simulink model "surgicalControl_Shared_memory_q_2015b"  (R2015b)
settings: Solver=FixedStepAuto  SolverMode=SingleTasking  StartTime=0.0  StopTime=inf  FixedStep=1/100  RelTol=1e-3
libraries: simulink x3, matlabGenericSHM_Block x1
settings Model: Creator=daniel  LastModifiedBy=Bogdan
settings DataIOCC: LimitDataPoints=off
settings DebuggingCC: AllowSymbolicDim=on  SFUnexpectedBacktrackingDiag=error  SFNoUnconditionalDefaultTransitionDiag=error
settings ModelReferenceCC: PropagateSignalLabelsOutOfModel=on
settings GRTTargetCC: TargetLangStandard=C99 (ISO)
settings ConfigComp: CovMetricSettings=dwe  CovHtmlReporting=off  CovSaveCumulativeToWorkspaceVar=off  CovSaveSingleToWorkspaceVar=off  CovModelRefEnable=Off  CovExternalEMLEnable=on

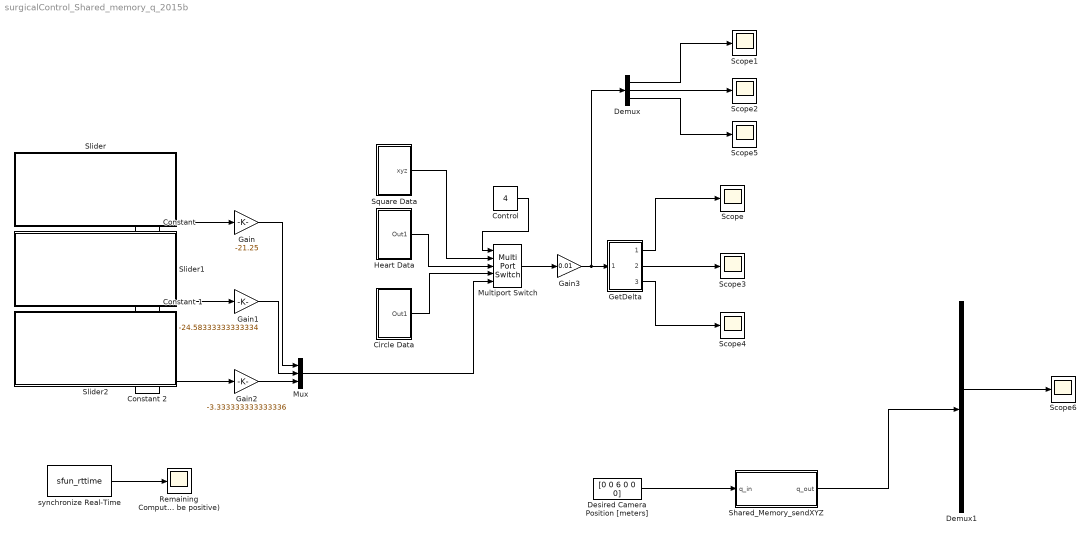
== system surgicalControl_Shared_memory_q_2015b ==
  " GetDelta " : Subsystem
  " Constant " : Constant
  " Constant 1" : Constant
  " Constant 2" : Constant
  "Circle Data " : Subsystem
  "Control " : Constant  Value=4
  Demux : Demux  Outputs=3
  Demux1 : Demux  Outputs=6
  Desired Camera Position [meters] : Constant  Value=[0 0 6 0 0 0]  OutDataTypeStr=single
  Gain : Gain  Gain=-21.25
  Gain1 : Gain  Gain=-24.58333333333334
  Gain2 : Gain  Gain=-3.333333333333336
  Gain3 : Gain  Gain=0.01
  "Heart Data " : Subsystem
  Multiport Switch : MultiPortSwitch  Inputs=4
  Mux : Mux  Inputs=3
  Remaining Computation Time (must be positive) : Scope
  Scope{,1..6} (7 alike) : Scope
  Shared_Memory_sendXYZ : Subsystem  mask{ID1=4}
  Slider : Subsystem  DialogController=hmiCreateDDGDialog  IsWebBlock=on  mask(MWDashboardBlock){webBlockId=4f94596f-dd6d-4e5e-bddc-7a8d913927f9, webBlockType=slider, ShowInLibBrowser=on, ShowInitialText=on, HMISrcModelName=surgicalControl_Shared_memory_q_2015b}
      mask prompts: webBlockId "WebBlock Id"; webBlockType "WebBlock Type"; HMISrcModelName "Source Model"
      mask help: SimulinkHMI:dialogs:SliderDialogDesc
      mask Help: helpview([docroot '/mapfiles/simulink.map'], 'hmi_slider')
      mask Display:
      | if strcmp(get_param(bdroot(gcb),'BlockDiagramType'), 'library')
      |     image([(matlabroot) '/toolbox/simulink/hmi/icons/Slider.png']);
      | end
  Slider1 : Subsystem  DialogController=hmiCreateDDGDialog  IsWebBlock=on  mask(MWDashboardBlock){webBlockId=8aa996ad-7cd4-40fc-9a04-6a85939aea5d, webBlockType=slider, ShowInLibBrowser=on, ShowInitialText=on, HMISrcModelName=surgicalControl_Shared_memory_q_2015b}
      mask prompts: webBlockId "WebBlock Id"; webBlockType "WebBlock Type"; HMISrcModelName "Source Model"
      mask help: SimulinkHMI:dialogs:SliderDialogDesc
      mask Help: helpview([docroot '/mapfiles/simulink.map'], 'hmi_slider')
      mask Display:
      | if strcmp(get_param(bdroot(gcb),'BlockDiagramType'), 'library')
      |     image([(matlabroot) '/toolbox/simulink/hmi/icons/Slider.png']);
      | end
  Slider2 : Subsystem  DialogController=hmiCreateDDGDialog  IsWebBlock=on  mask(MWDashboardBlock){webBlockId=1ddf6fd9-0225-4881-82ca-a25e179e2ab9, webBlockType=slider, ShowInLibBrowser=on, ShowInitialText=on, HMISrcModelName=surgicalControl_Shared_memory_q_2015b}
      mask prompts: webBlockId "WebBlock Id"; webBlockType "WebBlock Type"; HMISrcModelName "Source Model"
      mask help: SimulinkHMI:dialogs:SliderDialogDesc
      mask Help: helpview([docroot '/mapfiles/simulink.map'], 'hmi_slider')
      mask Display:
      | if strcmp(get_param(bdroot(gcb),'BlockDiagramType'), 'library')
      |     image([(matlabroot) '/toolbox/simulink/hmi/icons/Slider.png']);
      | end
  "Square Data " : Subsystem
  synchronize Real-Time : S-Function  FunctionName=sfun_rttime  Parameters=1  SFunctionDeploymentMode=off  EnableBusSupport=off
  wires:
  " GetDelta "/1(Out1) -> Scope/1
  " GetDelta "/2(Out2) -> Scope3/1
  " GetDelta "/3(Out3) -> Scope4/1
  Multiport Switch/1 -> Gain3/1
  "Square Data "/1(xyz) -> Multiport Switch/2
  "Control "/1 -> Multiport Switch/1
  " Constant "/1 -> Gain/1
  " Constant 1"/1 -> Gain1/1
  " Constant 2"/1 -> Gain2/1
  Gain/1 -> Mux/1
  Gain1/1 -> Mux/2
  Gain2/1 -> Mux/3
  Mux/1 -> Multiport Switch/5
  "Heart Data "/1(Out1) -> Multiport Switch/3
  "Circle Data "/1(Out1) -> Multiport Switch/4
  Demux/2 -> Scope2/1
  Demux/1 -> Scope1/1
  Demux/3 -> Scope5/1
  synchronize Real-Time/1 -> Remaining Computation Time (must be positive)/1
  Gain3/1 -> Demux/1, " GetDelta "/1(In1)
  Shared_Memory_sendXYZ/1(q_out) -> Demux1/1
  Desired Camera Position [meters]/1 -> Shared_Memory_sendXYZ/1(q_in)
  Demux1/3 -> Scope6/1

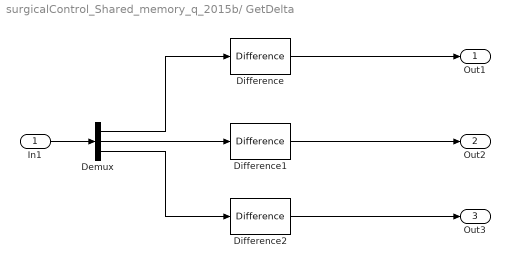
== system surgicalControl_Shared_memory_q_2015b/ GetDelta  ==
  In1 : Inport
  Demux : Demux  Outputs=3
  Difference : simulink/Discrete/Difference  ICPrevInput=0  OutMin=[]  OutMax=[]  OutDataType=fixdt(1, 16)  OutScaling=2^-10  DoSatur=off
  Difference1 : simulink/Discrete/Difference  ICPrevInput=0  OutMin=[]  OutMax=[]  OutDataType=fixdt(1, 16)  OutScaling=2^-10  DoSatur=off
  Difference2 : simulink/Discrete/Difference  ICPrevInput=0  OutMin=[]  OutMax=[]  OutDataType=fixdt(1, 16)  OutScaling=2^-10  DoSatur=off
  Out1 : Outport
  Out2 : Outport  Port=2
  Out3 : Outport  Port=3
  wires:
  Difference1/1 -> Out2/1
  Difference/1 -> Out1/1
  Difference2/1 -> Out3/1
  In1/1 -> Demux/1
  Demux/1 -> Difference/1
  Demux/2 -> Difference1/1
  Demux/3 -> Difference2/1

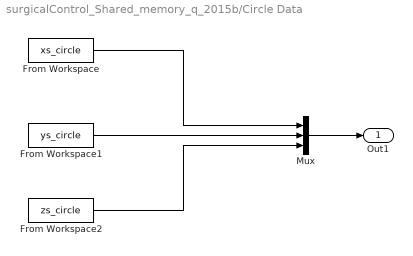
== system surgicalControl_Shared_memory_q_2015b/Circle Data  ==
  From Workspace : FromWorkspace  VariableName=xs_circle  SampleTime=1
  From Workspace1 : FromWorkspace  VariableName=ys_circle  SampleTime=1
  From Workspace2 : FromWorkspace  VariableName=zs_circle  SampleTime=1
  Mux : Mux  Inputs=3
  Out1 : Outport
  wires:
  From Workspace/1 -> Mux/1
  From Workspace2/1 -> Mux/3
  Mux/1 -> Out1/1
  From Workspace1/1 -> Mux/2

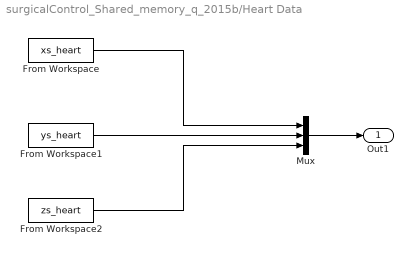
== system surgicalControl_Shared_memory_q_2015b/Heart Data  ==
  From Workspace : FromWorkspace  VariableName=xs_heart  SampleTime=1
  From Workspace1 : FromWorkspace  VariableName=ys_heart  SampleTime=1
  From Workspace2 : FromWorkspace  VariableName=zs_heart  SampleTime=1
  Mux : Mux  Inputs=3
  Out1 : Outport
  wires:
  From Workspace/1 -> Mux/1
  From Workspace2/1 -> Mux/3
  Mux/1 -> Out1/1
  From Workspace1/1 -> Mux/2

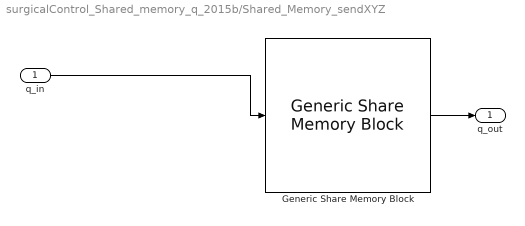
== system surgicalControl_Shared_memory_q_2015b/Shared_Memory_sendXYZ ==
  q_in : Inport
  Generic Share Memory Block : matlabGenericSHM_Block/Generic Share Memory Block  nombre='EyeRob'  dispositivo=ID1  vecE=[6]  vecS=[6]  tipoE=['f']  tipoS=['f']
  q_out : Outport
  wires:
  q_in/1 -> Generic Share Memory Block/1
  Generic Share Memory Block/1 -> q_out/1

== system surgicalControl_Shared_memory_q_2015b/Slider ==

== system surgicalControl_Shared_memory_q_2015b/Slider1 ==

== system surgicalControl_Shared_memory_q_2015b/Slider2 ==

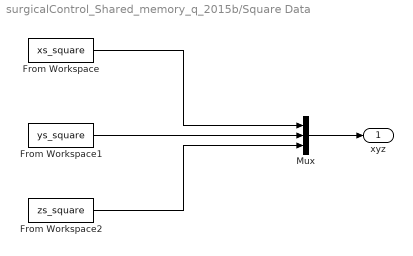
== system surgicalControl_Shared_memory_q_2015b/Square Data  ==
  From Workspace : FromWorkspace  VariableName=xs_square  SampleTime=1
  From Workspace1 : FromWorkspace  VariableName=ys_square  SampleTime=1
  From Workspace2 : FromWorkspace  VariableName=zs_square  SampleTime=1
  Mux : Mux  Inputs=3
  xyz : Outport
  wires:
  From Workspace/1 -> Mux/1
  From Workspace2/1 -> Mux/3
  Mux/1 -> xyz/1
  From Workspace1/1 -> Mux/2
